simulink model "vitesse_disc"  (R2020a)
settings: Solver=VariableStepAuto  StartTime=0.0  StopTime=0.05  RelTol=1e-3
values from neighbouring files (symbols this model uses):
  a20 = -a21    (= -0.007212)    [be_trot.m]
  a21 = 2*Ti2    (= 0.007212)    [be_trot.m]
  b20 = Te2 - 2*Tc2    (= -0.03164)    [be_trot.m]
  b21 = Te2 + 2*Tc2    (= 0.03204)    [be_trot.m]
  Kb = (7.1875/0.5)/(0.233)    (= 61.69527897)    [be_trot.m]
  KT = 3.3/20    (= 0.165)    [be_trot.m]
  Te2 = 1/5000    (= 0.0002)    [be_trot.m]
settings Model: Creator=lagrost  LastModifiedBy=gauthero

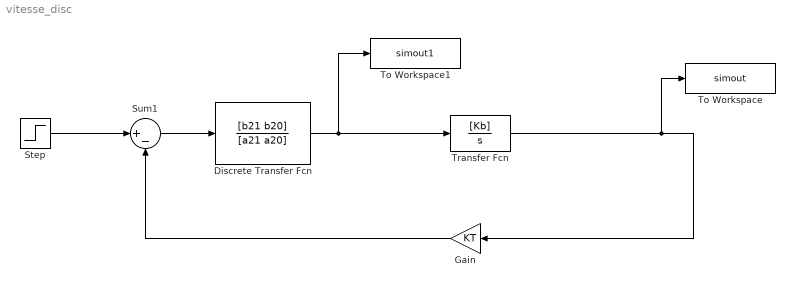
== system vitesse_disc ==
  Discrete Transfer Fcn : DiscreteTransferFcn  Numerator=[b21 b20]  Denominator=[a21 a20]  SampleTime=Te2
  Gain : Gain  Gain=KT
  Step : Step  Time=0  SampleTime=0
  Sum1 : Sum  Inputs=|+-
  To Workspace : ToWorkspace  VariableName=simout  SaveFormat=Timeseries  SampleTime=-1
  To Workspace1 : ToWorkspace  VariableName=simout1  SaveFormat=Timeseries  SampleTime=-1
  Transfer Fcn : TransferFcn  Numerator=[Kb]  Denominator=[1 0]
  wires:
  Step/1 -> Sum1/1
  Sum1/1 -> Discrete Transfer Fcn/1
  Transfer Fcn/1 -> Gain/1, To Workspace/1
  Discrete Transfer Fcn/1 -> To Workspace1/1, Transfer Fcn/1
  Gain/1 -> Sum1/2
